simulink model "quadraturmischer"  (Simulink 7.7)
settings: Solver=VariableStepDiscrete  StartTime=0.0  StopTime=simulationTime  RelTol=1e-3
values from neighbouring files (symbols this model uses):
  f0 = 1    [Correlation_kreuz.m]    (also in InterpolateSignalVector.m; fft_whyFactorL.m = 0; fourier_reihe_vs_trans.m = 0.2; quadraturmixer_config.m = 300)
  phaseCos = 90*(180/pi)    (= 5156.62015618)    [quadraturmixer_config.m]
  phaseSin = 0    [quadraturmixer_config.m]
  sampleTime = Ts    (= 0.0005)    [quadraturmixer_config.m]
  Ts = Tsam*Fsam    (= 1)    [BPSK_selfmade.m]    (also in FFT_iFFT.m = 0.0002; InterpolateSignalVector.m = 0.0025; QPSK_constellation.m; correlationSample.m)
undefined symbols (not defined in the file or in its folder): dfilt, fdesignblkfcn, gcbh
libraries: dsparch4 x1
settings Model: Creator=mainster  LastModifiedBy=mainster

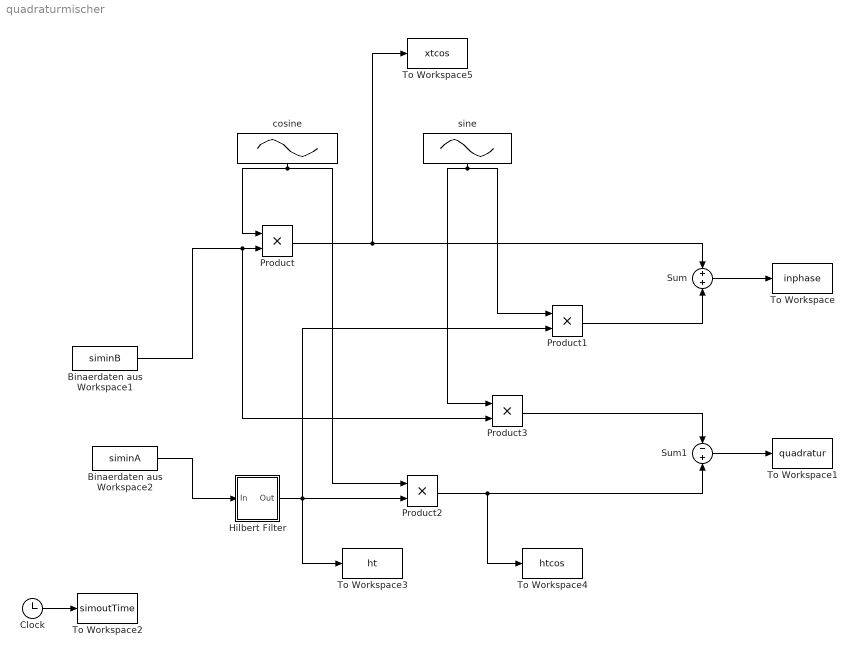
== system quadraturmischer ==
  Binaerdaten aus Workspace1 : FromWorkspace  VariableName=siminB  SampleTime=sampleTime
  Binaerdaten aus Workspace2 : FromWorkspace  VariableName=siminA  SampleTime=sampleTime
  Clock : Clock
  Hilbert Filter : Subsystem  DialogController=fdesignblkfcn  DialogControllerArgs=DataTag1  InitFcn=fdesignblkfcn(gcbh, {'InitFcn'});
      settings: CopyFcn=fdesignblkfcn(gcbh, {'CopyFcn'});
      mask Type: Hilbert Filter
      mask Description: Design a hilbert filter filter
      mask Help: helpview(mapfilelocation('dsp'), 'dsphilbertfilter');
      mask Display: disp('Hilbert')
  Product{,1..3} (4 alike) : Product  SampleTime=Ts  RndMeth=Zero
  Sum : Sum  SampleTime=Ts
  Sum1 : Sum  Inputs=-+  SampleTime=Ts
  To Workspace : ToWorkspace  VariableName=inphase  SampleTime=Ts  SaveFormat=Structure
  To Workspace1 : ToWorkspace  VariableName=quadratur  SampleTime=Ts  SaveFormat=Structure
  To Workspace2 : ToWorkspace  VariableName=simoutTime  SampleTime=-1  SaveFormat=Structure
  To Workspace3 : ToWorkspace  VariableName=ht  SampleTime=Ts  SaveFormat=Structure
  To Workspace4 : ToWorkspace  VariableName=htcos  SampleTime=Ts  SaveFormat=Structure
  To Workspace5 : ToWorkspace  VariableName=xtcos  SampleTime=Ts  SaveFormat=Structure
  cosine : Sin  Frequency=2*pi*f0  Phase=phaseCos  SampleTime=Ts
  sine : Sin  Frequency=2*pi*f0  Phase=phaseSin  SampleTime=Ts
  wires:
  Binaerdaten aus Workspace1/1 -> Product/2, Product3/2
  Hilbert Filter/1(Out) -> Product2/2, Product1/2, To Workspace3/1
  Product/1 -> Sum/1, To Workspace5/1
  Product1/1 -> Sum/2
  Product3/1 -> Sum1/1
  Product2/1 -> Sum1/2, To Workspace4/1
  sine/1 -> Product1/1, Product3/1
  cosine/1 -> Product/1, Product2/1
  Sum1/1 -> To Workspace1/1
  Sum/1 -> To Workspace/1
  Clock/1 -> To Workspace2/1
  Binaerdaten aus Workspace2/1 -> Hilbert Filter/1(In)

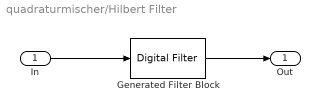
== system quadraturmischer/Hilbert Filter ==
  In : Inport
  Generated Filter Block : dsparch4/Digital Filter  Tag=BlockMethodSubSystem  TypePopup=FIR (all zeros)  IIRFiltStruct=Direct form II transposed  AllPoleFiltStruct=Direct form  FIRFiltStruct=Direct form  CoeffSource=Specify via dialog  NumCoeffs=[-0.0264498582597914 -0.00578355491829027 -0.0165722619033485 -0.00953905611319827 -0.0224613905350716 -0.014999256435126 -0.0303239670747386 -0.023012528163449 -0.0414293158216551 -0.0357628289392783 -0.0591175238175318 -0.0590346854108087 -0.0944599066521764 -0.117398302041723 -0.217977189936103 -0.628693537472792 0.628693537472792 0.217977189936103 0.117398302041723 0.0944599066521764 0.0590346854108087 0.0591175238175318 0.0357628289392783 0.0414293158216551 0.023012528163449 0.0303239670747386 0.014999256435126 0.0224613905350716 0.00953905611319827 0.0165722619033485 0.00578355491829027 0.0264498582597914]  DenCoeffs=[1 0.1]  BiQuadCoeffs=[1 0.3 0.4 1 0.1 0.2]  LatticeCoeffs=[0.2 0.4]  denIgnore=on  FiltPerSampPopup=One filter per frame  IC=0  ICnum=0  ICden=0  roundingMode=Floor  overflowMode=off  ScaleValues=1  scaleValueFracLength=14  stageInFracLength=15  stageOutFracLength=15  FilterSource=Specify via dialog  dfiltObjectName=dfilt.dffir([1 2 1])  InputProcessing=Columns as channels (frame based)
  Out : Outport
  wires:
  Generated Filter Block/1 -> Out/1
  In/1 -> Generated Filter Block/1
